simulink library "aerosimlib"  (Simulink 5.0)
values from neighbouring files (symbols this model uses):
  stdatm = [0 100 200 300 400 500 600 700 800 900 1000 1100 ... (4305 elements, 861x5)]    [stdatm.mat]
undefined symbols (not defined in the file or in its folder): AlphaBnd, b, BetaBnd, CDda, CDde, CDdf, CDdr, CDM, CDmin, CGempty, CGgross, CL0, CLa, CLalphadot, Clbeta, Clda, CLde, CLdf, Cldr, CLM, CLmind, Clp, CLq, Clr, Cm0, Cma, Cmalphadot, Cmde, Cmdf, CmM, Cmq, Cnbeta, Cnda, Cndr, Cnp, Cnr, CP, CT, CYbeta, CYda, CYdr, CYp, CYr, Displacement, dmy, Engine, EulerIni, FuelFlow, FuelIni, J, Jempty, Jeng, Jgross, Jprop, MAC, MAP, MAPLim, MassIni, MaxPower, mempty ... (+25)
libraries: aerosimlib x350, simulink3 x41
(part 9 of 10)

== system aerosimlib/FlightGear-Compatible/Complete Aircraft/CESSNA-182/Aerodynamics/Roll ==
  Control : Inport  PortDimensions=[4 1]
  WindAxesVel : Inport  Port=2  PortDimensions=[3 1]
  AngularRates : Inport  Port=3  PortDimensions=[3 1]
  2 : Gain  Gain=2  SaturateOnIntegerOverflow=on
  Cl aileron : Subsystem  BlockChoice=Value
      link override Value: Value=AC.Aerodynamics.Roll.ClDa
      settings: AttributesFormatString=%<BlockChoice>  TemplateBlock=aerosimlib/FlightGear-Compatible/Aerodynamics/Coefficient  MemberBlocks=Table,Value,Vector
  Cl beta : Subsystem  BlockChoice=Table
      link override Table: Table=AC.Aerodynamics.Roll.Clb
      link override Value: Value=AC.Aerodynamics.Lift.Basic.kCLge
      link override Vector: Vector=AC.Aerodynamics.Roll.Clb
      settings: AttributesFormatString=%<BlockChoice>  TemplateBlock=aerosimlib/FlightGear-Compatible/Aerodynamics/Coefficient  MemberBlocks=Table,Value,Vector
  Cl rudder : Subsystem  BlockChoice=Value
      link override Value: Value=AC.Aerodynamics.Roll.ClDr
      settings: AttributesFormatString=%<BlockChoice>  TemplateBlock=aerosimlib/FlightGear-Compatible/Aerodynamics/Coefficient  MemberBlocks=Table,Value,Vector
  Cl*b/(2V) : Product  Inputs=**/  SaturateOnIntegerOverflow=on  InputSameDT=on
  Clp : Subsystem  BlockChoice=Vector
      link override Value: Value=AC.Aerodynamics.Roll.Clp
      link override Vector: Vector=AC.Aerodynamics.Roll.Clp
      settings: AttributesFormatString=%<BlockChoice>  TemplateBlock=aerosimlib/FlightGear-Compatible/Aerodynamics/Coefficient  MemberBlocks=Table,Value,Vector
  Clp*p : Product  SaturateOnIntegerOverflow=on  InputSameDT=on
  Clr : Subsystem  BlockChoice=Vector
      link override Value: Value=AC.Aerodynamics.Side.CYdr
      link override Vector: Vector=AC.Aerodynamics.Roll.Clr
      settings: AttributesFormatString=%<BlockChoice>  TemplateBlock=aerosimlib/FlightGear-Compatible/Aerodynamics/Coefficient  MemberBlocks=Table,Value,Vector
  Clr*r : Product  SaturateOnIntegerOverflow=on  InputSameDT=on
  Demux : Demux
  Demux1 : Demux  Outputs=3
  Demux3 : Demux  Outputs=3
  Sum : Sum  SaturateOnIntegerOverflow=on  InputSameDT=on
  Sum1 : Sum  Inputs=++++  SaturateOnIntegerOverflow=on  InputSameDT=on
  Terminator2 : Terminator
  Terminator3 : Terminator
  Terminator4 : Terminator
  Wing span : Constant  Value=AC.Metrics.WingSpan
  Cl : Outport
  wires:
  Demux3/3 -> Clr*r/2
  Demux3/1 -> Clp*p/2
  Clp*p/1 -> Sum/1
  Clr*r/1 -> Sum/2
  Clr/1(Coeff) -> Clr*r/1
  Clp/1(Coeff) -> Clp*p/1
  Sum1/1 -> Cl/1
  AngularRates/1 -> Demux3/1
  Control/1 -> Demux/1
  WindAxesVel/1 -> Demux1/1
  Wing span/1 -> Cl*b/(2V)/2
  2/1 -> Cl*b/(2V)/3
  Sum/1 -> Cl*b/(2V)/1
  Demux1/1 -> 2/1
  Demux1/2 -> Cl beta/1(RowParam)
  Demux/3 -> Cl aileron/1(RowParam)
  Demux/4 -> Cl rudder/1(RowParam)
  Demux3/2 -> Terminator4/1
  Demux1/3 -> Clr/1(RowParam), Clp/1(RowParam), Cl beta/2(ColParam)
  Demux/1 -> Terminator2/1
  Demux/2 -> Terminator3/1
  Cl beta/1(Coeff) -> Sum1/1
  Cl aileron/1(Coeff) -> Sum1/2
  Cl rudder/1(Coeff) -> Sum1/3
  Cl*b/(2V)/1 -> Sum1/4

== system aerosimlib/FlightGear-Compatible/Complete Aircraft/CESSNA-182/Aerodynamics/Side ==
  Control : Inport  PortDimensions=[4 1]
  WindAxesVel : Inport  Port=2  PortDimensions=[3 1]
  AngularRates : Inport  Port=3  PortDimensions=[3 1]
  2 : Gain  Gain=2  SaturateOnIntegerOverflow=on
  CY aileron : Subsystem  BlockChoice=Value
      link override Value: Value=AC.Aerodynamics.Side.CYDa
      settings: AttributesFormatString=%<BlockChoice>  TemplateBlock=aerosimlib/FlightGear-Compatible/Aerodynamics/Coefficient  MemberBlocks=Table,Value,Vector
  CY beta : Subsystem  BlockChoice=Vector
      link override Value: Value=AC.Aerodynamics.Lift.Basic.kCLge
      link override Vector: Vector=AC.Aerodynamics.Side.CYb
      settings: AttributesFormatString=%<BlockChoice>  TemplateBlock=aerosimlib/FlightGear-Compatible/Aerodynamics/Coefficient  MemberBlocks=Table,Value,Vector
  CY rudder : Subsystem  BlockChoice=Value
      link override Value: Value=AC.Aerodynamics.Side.CYDr
      settings: AttributesFormatString=%<BlockChoice>  TemplateBlock=aerosimlib/FlightGear-Compatible/Aerodynamics/Coefficient  MemberBlocks=Table,Value,Vector
  CY*b/(2V) : Product  Inputs=**/  SaturateOnIntegerOverflow=on  InputSameDT=on
  CYb*b : Product  SaturateOnIntegerOverflow=on  InputSameDT=on
  CYp : Subsystem  BlockChoice=Vector
      link override Value: Value=AC.Aerodynamics.Side.CYp
      link override Vector: Vector=AC.Aerodynamics.Side.CYp
      settings: AttributesFormatString=%<BlockChoice>  TemplateBlock=aerosimlib/FlightGear-Compatible/Aerodynamics/Coefficient  MemberBlocks=Table,Value,Vector
  CYp*p : Product  SaturateOnIntegerOverflow=on  InputSameDT=on
  CYr : Subsystem  BlockChoice=Vector
      link override Value: Value=AC.Aerodynamics.Side.CYr
      link override Vector: Vector=AC.Aerodynamics.Side.CYr
      settings: AttributesFormatString=%<BlockChoice>  TemplateBlock=aerosimlib/FlightGear-Compatible/Aerodynamics/Coefficient  MemberBlocks=Table,Value,Vector
  CYr*r : Product  SaturateOnIntegerOverflow=on  InputSameDT=on
  Demux : Demux
  Demux1 : Demux  Outputs=3
  Demux3 : Demux  Outputs=3
  Sum : Sum  SaturateOnIntegerOverflow=on  InputSameDT=on
  Sum1 : Sum  Inputs=++++  SaturateOnIntegerOverflow=on  InputSameDT=on
  Terminator2 : Terminator
  Terminator3 : Terminator
  Terminator4 : Terminator
  Wing span : Constant  Value=AC.Metrics.WingSpan
  CY : Outport
  wires:
  Demux3/3 -> CYr*r/2
  Demux3/1 -> CYp*p/2
  CYr*r/1 -> Sum/2
  CYr/1(Coeff) -> CYr*r/1
  CYp*p/1 -> Sum/1
  CYp/1(Coeff) -> CYp*p/1
  Demux1/2 -> CYb*b/2
  CYb*b/1 -> Sum1/1
  CY beta/1(Coeff) -> CYb*b/1
  CY*b/(2V)/1 -> Sum1/4
  CY rudder/1(Coeff) -> Sum1/3
  CY aileron/1(Coeff) -> Sum1/2
  Demux/2 -> Terminator3/1
  Demux/1 -> Terminator2/1
  Demux1/3 -> CYr/1(RowParam), CYp/1(RowParam), CY beta/1(RowParam)
  Demux3/2 -> Terminator4/1
  Demux/4 -> CY rudder/1(RowParam)
  Demux/3 -> CY aileron/1(RowParam)
  Demux1/1 -> 2/1
  Sum/1 -> CY*b/(2V)/1
  2/1 -> CY*b/(2V)/3
  Wing span/1 -> CY*b/(2V)/2
  WindAxesVel/1 -> Demux1/1
  Control/1 -> Demux/1
  AngularRates/1 -> Demux3/1
  Sum1/1 -> CY/1

== system aerosimlib/FlightGear-Compatible/Complete Aircraft/CESSNA-182/Aerodynamics/Yaw ==
  Control : Inport  PortDimensions=[4 1]
  WindAxesVel : Inport  Port=2  PortDimensions=[3 1]
  AngularRates : Inport  Port=3  PortDimensions=[3 1]
  2 : Gain  Gain=2  SaturateOnIntegerOverflow=on
  Cn aileron : Subsystem  BlockChoice=Vector
      link override Value: Value=AC.Aerodynamics.Yaw.Cnda
      link override Vector: Vector=AC.Aerodynamics.Yaw.CnDa
      settings: AttributesFormatString=%<BlockChoice>  TemplateBlock=aerosimlib/FlightGear-Compatible/Aerodynamics/Coefficient  MemberBlocks=Table,Value,Vector
  Cn beta : Subsystem  BlockChoice=Vector
      link override Value: Value=AC.Aerodynamics.Lift.Basic.kCLge
      link override Vector: Vector=AC.Aerodynamics.Yaw.Cnb
      settings: AttributesFormatString=%<BlockChoice>  TemplateBlock=aerosimlib/FlightGear-Compatible/Aerodynamics/Coefficient  MemberBlocks=Table,Value,Vector
  Cn rudder : Subsystem  BlockChoice=Vector
      link override Value: Value=AC.Aerodynamics.Yaw.Cndr
      link override Vector: Vector=AC.Aerodynamics.Yaw.CnDr
      settings: AttributesFormatString=%<BlockChoice>  TemplateBlock=aerosimlib/FlightGear-Compatible/Aerodynamics/Coefficient  MemberBlocks=Table,Value,Vector
  Cn*b/(2V) : Product  Inputs=**/  SaturateOnIntegerOverflow=on  InputSameDT=on
  Cnb*b{,1..4} (5 alike) : Product  SaturateOnIntegerOverflow=on  InputSameDT=on
  Cnp : Subsystem  BlockChoice=Vector
      link override Value: Value=AC.Aerodynamics.Yaw.Cnp
      link override Vector: Vector=AC.Aerodynamics.Yaw.Cnp
      settings: AttributesFormatString=%<BlockChoice>  TemplateBlock=aerosimlib/FlightGear-Compatible/Aerodynamics/Coefficient  MemberBlocks=Table,Value,Vector
  Cnr : Subsystem  BlockChoice=Vector
      link override Value: Value=AC.Aerodynamics.Yaw.Cnr
      link override Vector: Vector=AC.Aerodynamics.Yaw.Cnr
      settings: AttributesFormatString=%<BlockChoice>  TemplateBlock=aerosimlib/FlightGear-Compatible/Aerodynamics/Coefficient  MemberBlocks=Table,Value,Vector
  Demux : Demux
  Demux1 : Demux  Outputs=3
  Demux3 : Demux  Outputs=3
  Sum : Sum  SaturateOnIntegerOverflow=on  InputSameDT=on
  Sum1 : Sum  Inputs=++++  SaturateOnIntegerOverflow=on  InputSameDT=on
  Terminator2 : Terminator
  Terminator3 : Terminator
  Terminator4 : Terminator
  Wing span : Constant  Value=AC.Metrics.WingSpan
  Cn : Outport
  wires:
  Demux3/3 -> Cnb*b4/2
  Demux3/1 -> Cnb*b3/2
  Demux/4 -> Cnb*b2/2
  Demux/3 -> Cnb*b1/2
  Cnb*b2/1 -> Sum1/3
  Cnb*b1/1 -> Sum1/2
  Cnb*b3/1 -> Sum/1
  Cnb*b4/1 -> Sum/2
  Cnr/1(Coeff) -> Cnb*b4/1
  Cnp/1(Coeff) -> Cnb*b3/1
  Cn rudder/1(Coeff) -> Cnb*b2/1
  Cn aileron/1(Coeff) -> Cnb*b1/1
  Demux1/2 -> Cnb*b/2
  Cn beta/1(Coeff) -> Cnb*b/1
  Cnb*b/1 -> Sum1/1
  Cn*b/(2V)/1 -> Sum1/4
  Demux/2 -> Terminator3/1
  Demux/1 -> Terminator2/1
  Demux1/3 -> Cnp/1(RowParam), Cnr/1(RowParam), Cn rudder/1(RowParam), Cn aileron/1(RowParam), Cn beta/1(RowParam)
  Demux3/2 -> Terminator4/1
  Demux1/1 -> 2/1
  Sum/1 -> Cn*b/(2V)/1
  2/1 -> Cn*b/(2V)/3
  Wing span/1 -> Cn*b/(2V)/2
  WindAxesVel/1 -> Demux1/1
  Control/1 -> Demux/1
  AngularRates/1 -> Demux3/1
  Sum1/1 -> Cn/1

== system aerosimlib/FlightGear-Compatible/Complete Aircraft/CESSNA-310/Aerodynamics/Drag ==
  Control : Inport  PortDimensions=[4 1]
  WindAxesVel : Inport  Port=2  PortDimensions=[3 1]
  Gear : Inport  Port=3  PortDimensions=1
  CD alpha : Subsystem  BlockChoice=Vector
      link override Table: Table=AC.Aerodynamics.Drag.Basic.CDwbh
      link override Value: Value=AC.Aerodynamics.Lift.Basic.kCLge
      link override Vector: Vector=AC.Aerodynamics.Drag.CDalpha
      settings: AttributesFormatString=%<BlockChoice>  TemplateBlock=aerosimlib/FlightGear-Compatible/Aerodynamics/Coefficient  MemberBlocks=Table,Value,Vector
  CD beta : Subsystem  BlockChoice=Value
      link override Value: Value=AC.Aerodynamics.Drag.CDbeta
      settings: AttributesFormatString=%<BlockChoice>  TemplateBlock=aerosimlib/FlightGear-Compatible/Aerodynamics/Coefficient  MemberBlocks=Table,Value,Vector
  CD elevator : Subsystem  BlockChoice=Value
      link override Value: Value=AC.Aerodynamics.Drag.CDDe
      settings: AttributesFormatString=%<BlockChoice>  TemplateBlock=aerosimlib/FlightGear-Compatible/Aerodynamics/Coefficient  MemberBlocks=Table,Value,Vector
  CD flap : Subsystem  BlockChoice=Vector
      link override Table: Table=AC.Aerodynamics.Drag.CDDf
      link override Value: Value=AC.Aerodynamics.Lift.Basic.kCLge
      link override Vector: Vector=AC.Aerodynamics.Drag.CDDf
      settings: AttributesFormatString=%<BlockChoice>  TemplateBlock=aerosimlib/FlightGear-Compatible/Aerodynamics/Coefficient  MemberBlocks=Table,Value,Vector
  CD gear : Subsystem  BlockChoice=Value
      link override Value: Value=AC.Aerodynamics.Drag.CDgear
      settings: AttributesFormatString=%<BlockChoice>  TemplateBlock=aerosimlib/FlightGear-Compatible/Aerodynamics/Coefficient  MemberBlocks=Table,Value,Vector
  CDo : Constant  Value=AC.Aerodynamics.Drag.CDo.Data
  Demux : Demux
  Demux1 : Demux  Outputs=3
  Sum : Sum  SaturateOnIntegerOverflow=on  InputSameDT=on
  Sum1 : Sum  Inputs=+++++  SaturateOnIntegerOverflow=on  InputSameDT=on
  Terminator : Terminator
  Terminator1 : Terminator
  Terminator5 : Terminator
  CD : Outport
  wires:
  Gear/1 -> CD gear/1(RowParam)
  CD gear/1(Coeff) -> Sum1/5
  Demux/2 -> CD elevator/1(RowParam)
  WindAxesVel/1 -> Demux1/1
  Control/1 -> Demux/1
  Demux/3 -> Terminator/1
  Demux/4 -> Terminator1/1
  Demux1/3 -> CD alpha/1(RowParam)
  CD alpha/1(Coeff) -> Sum/1
  CD flap/1(Coeff) -> Sum/2
  Sum/1 -> Sum1/1
  CDo/1 -> Sum1/2
  CD elevator/1(Coeff) -> Sum1/3
  Sum1/1 -> CD/1
  Demux1/1 -> Terminator5/1
  Demux1/2 -> CD beta/1(RowParam)
  Demux/1 -> CD flap/1(RowParam)
  CD beta/1(Coeff) -> Sum1/4

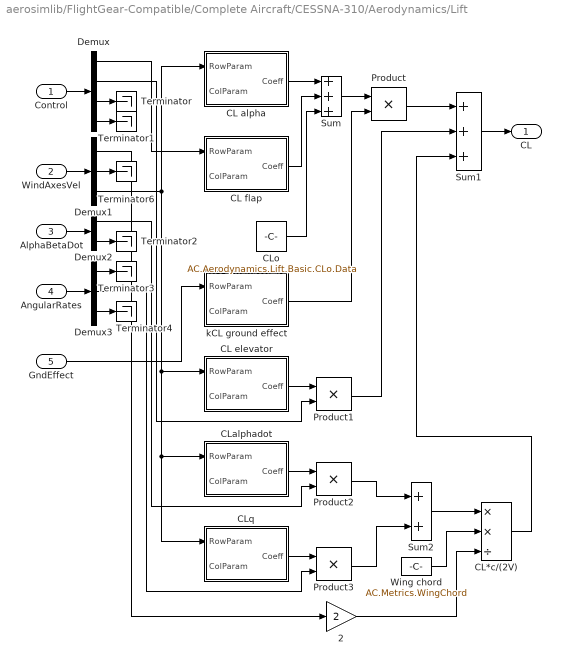
== system aerosimlib/FlightGear-Compatible/Complete Aircraft/CESSNA-310/Aerodynamics/Lift ==
  Control : Inport  PortDimensions=[4 1]
  WindAxesVel : Inport  Port=2  PortDimensions=[3 1]
  AlphaBetaDot : Inport  Port=3  PortDimensions=[2 1]
  AngularRates : Inport  Port=4  PortDimensions=[3 1]
  GndEffect : Inport  Port=5  PortDimensions=1
  2 : Gain  Gain=2  SaturateOnIntegerOverflow=on
  CL alpha : Subsystem  BlockChoice=Vector
      link override Table: Table=AC.Aerodynamics.Lift.Basic.CLalpha
      link override Value: Value=AC.Aerodynamics.Lift.Basic.kCLge
      link override Vector: Vector=AC.Aerodynamics.Lift.Basic.CLalpha
      settings: AttributesFormatString=%<BlockChoice>  TemplateBlock=aerosimlib/FlightGear-Compatible/Aerodynamics/Coefficient  MemberBlocks=Table,Value,Vector
  CL elevator : Subsystem  BlockChoice=Vector
      link override Value: Value=AC.Aerodynamics.Lift.CLDe
      link override Vector: Vector=AC.Aerodynamics.Lift.CLDe
      settings: AttributesFormatString=%<BlockChoice>  TemplateBlock=aerosimlib/FlightGear-Compatible/Aerodynamics/Coefficient  MemberBlocks=Table,Value,Vector
  CL flap : Subsystem  BlockChoice=Vector
      link override Value: Value=AC.Aerodynamics.Lift.Basic.kCLge
      link override Vector: Vector=AC.Aerodynamics.Lift.Basic.CLDf
      settings: AttributesFormatString=%<BlockChoice>  TemplateBlock=aerosimlib/FlightGear-Compatible/Aerodynamics/Coefficient  MemberBlocks=Table,Value,Vector
  CL*c/(2V) : Product  Inputs=**/  SaturateOnIntegerOverflow=on  InputSameDT=on
  CLalphadot : Subsystem  BlockChoice=Vector
      link override Value: Value=AC.Aerodynamics.Lift.CLadot
      link override Vector: Vector=AC.Aerodynamics.Lift.CLadot
      settings: AttributesFormatString=%<BlockChoice>  TemplateBlock=aerosimlib/FlightGear-Compatible/Aerodynamics/Coefficient  MemberBlocks=Table,Value,Vector
  CLo : Constant  Value=AC.Aerodynamics.Lift.Basic.CLo.Data
  CLq : Subsystem  BlockChoice=Vector
      link override Value: Value=AC.Aerodynamics.Lift.CLq
      link override Vector: Vector=AC.Aerodynamics.Lift.CLq
      settings: AttributesFormatString=%<BlockChoice>  TemplateBlock=aerosimlib/FlightGear-Compatible/Aerodynamics/Coefficient  MemberBlocks=Table,Value,Vector
  Demux : Demux
  Demux1 : Demux  Outputs=3
  Demux2 : Demux  Outputs=2
  Demux3 : Demux  Outputs=3
  Product{,1..3} (4 alike) : Product  SaturateOnIntegerOverflow=on  InputSameDT=on
  Sum : Sum  Inputs=+++  SaturateOnIntegerOverflow=on  InputSameDT=on
  Sum1 : Sum  Inputs=+++  SaturateOnIntegerOverflow=on  InputSameDT=on
  Sum2 : Sum  SaturateOnIntegerOverflow=on  InputSameDT=on
  Terminator{,1..4,6} (6 alike) : Terminator
  Wing chord : Constant  Value=AC.Metrics.WingChord
  kCL ground effect : Subsystem  BlockChoice=Vector
      link override Value: Value=AC.Aerodynamics.Lift.Basic.kCLge
      link override Vector: Vector=AC.Aerodynamics.Lift.Basic.kCLge
      settings: AttributesFormatString=%<BlockChoice>  TemplateBlock=aerosimlib/FlightGear-Compatible/Aerodynamics/Coefficient  MemberBlocks=Table,Value,Vector
  CL : Outport
  wires:
  Demux3/2 -> Product3/2
  Demux2/1 -> Product2/2
  Demux/2 -> Product1/2
  Product1/1 -> Sum1/2
  Product2/1 -> Sum2/1
  Product3/1 -> Sum2/2
  CLq/1(Coeff) -> Product3/1
  CLalphadot/1(Coeff) -> Product2/1
  CL elevator/1(Coeff) -> Product1/1
  CLo/1 -> Sum/3
  CL*c/(2V)/1 -> Sum1/3
  Sum2/1 -> CL*c/(2V)/1
  Wing chord/1 -> CL*c/(2V)/2
  2/1 -> CL*c/(2V)/3
  GndEffect/1 -> kCL ground effect/1(RowParam)
  Demux1/2 -> Terminator6/1
  Demux1/1 -> 2/1
  Sum1/1 -> CL/1
  Product/1 -> Sum1/1
  kCL ground effect/1(Coeff) -> Product/2
  Sum/1 -> Product/1
  CL flap/1(Coeff) -> Sum/2
  CL alpha/1(Coeff) -> Sum/1
  Demux3/3 -> Terminator4/1
  Demux3/1 -> Terminator3/1
  Demux2/2 -> Terminator2/1
  Demux1/3 -> CLq/1(RowParam), CLalphadot/1(RowParam), CL elevator/1(RowParam), CL alpha/1(RowParam)
  Demux/4 -> Terminator1/1
  Demux/3 -> Terminator/1
  Demux/1 -> CL flap/1(RowParam)
  AngularRates/1 -> Demux3/1
  AlphaBetaDot/1 -> Demux2/1
  Control/1 -> Demux/1
  WindAxesVel/1 -> Demux1/1

== system aerosimlib/FlightGear-Compatible/Complete Aircraft/CESSNA-310/Aerodynamics/Pitch ==
  Control : Inport  PortDimensions=[4 1]
  WindAxesVel : Inport  Port=2  PortDimensions=[3 1]
  AlphaBetaDot : Inport  Port=3  PortDimensions=[2 1]
  AngularRates : Inport  Port=4  PortDimensions=[3 1]
  2 : Gain  Gain=2  SaturateOnIntegerOverflow=on
  Cm alpha : Subsystem  BlockChoice=Value
      link override Table: Table=AC.Aerodynamics.Lift.Basic.CLwbh
      link override Value: Value=AC.Aerodynamics.Pitch.Cmalpha
      link override Vector: Vector=AC.Aerodynamics.Pitch.Cmalpha
      settings: AttributesFormatString=%<BlockChoice>  TemplateBlock=aerosimlib/FlightGear-Compatible/Aerodynamics/Coefficient  MemberBlocks=Table,Value,Vector
  Cm elevator : Subsystem  BlockChoice=Value
      link override Value: Value=AC.Aerodynamics.Pitch.CmDe
      link override Vector: Vector=AC.Aerodynamics.Pitch.CmDe
      settings: AttributesFormatString=%<BlockChoice>  TemplateBlock=aerosimlib/FlightGear-Compatible/Aerodynamics/Coefficient  MemberBlocks=Table,Value,Vector
  Cm flap : Subsystem  BlockChoice=Vector
      link override Value: Value=AC.Aerodynamics.Lift.Basic.kCLge
      link override Vector: Vector=AC.Aerodynamics.Pitch.CmDf
      settings: AttributesFormatString=%<BlockChoice>  TemplateBlock=aerosimlib/FlightGear-Compatible/Aerodynamics/Coefficient  MemberBlocks=Table,Value,Vector
  Cm*c/(2V) : Product  Inputs=**/  SaturateOnIntegerOverflow=on  InputSameDT=on
  Cmalphadot : Subsystem  BlockChoice=Value
      link override Value: Value=AC.Aerodynamics.Pitch.Cmadot
      link override Vector: Vector=AC.Aerodynamics.Pitch.Cmadot
      settings: AttributesFormatString=%<BlockChoice>  TemplateBlock=aerosimlib/FlightGear-Compatible/Aerodynamics/Coefficient  MemberBlocks=Table,Value,Vector
  Cmo : Constant  Value=AC.Aerodynamics.Pitch.Cmo.Data
  Cmq : Subsystem  BlockChoice=Value
      link override Value: Value=AC.Aerodynamics.Pitch.Cmq
      link override Vector: Vector=AC.Aerodynamics.Pitch.Cmq
      settings: AttributesFormatString=%<BlockChoice>  TemplateBlock=aerosimlib/FlightGear-Compatible/Aerodynamics/Coefficient  MemberBlocks=Table,Value,Vector
  Demux : Demux
  Demux1 : Demux  Outputs=3
  Demux2 : Demux  Outputs=2
  Demux3 : Demux  Outputs=3
  Sum1 : Sum  Inputs=+++++  SaturateOnIntegerOverflow=on  InputSameDT=on
  Sum2 : Sum  SaturateOnIntegerOverflow=on  InputSameDT=on
  Terminator{,1..4,6} (6 alike) : Terminator
  Wing chord : Constant  Value=AC.Metrics.WingChord
  Cm : Outport
  wires:
  Cm elevator/1(Coeff) -> Sum1/4
  Cm alpha/1(Coeff) -> Sum1/1
  Cm*c/(2V)/1 -> Sum1/5
  Cmo/1 -> Sum1/3
  Cm flap/1(Coeff) -> Sum1/2
  Demux1/3 -> Cm alpha/1(RowParam)
  Demux1/1 -> 2/1
  Demux/1 -> Cm flap/1(RowParam)
  WindAxesVel/1 -> Demux1/1
  Control/1 -> Demux/1
  AlphaBetaDot/1 -> Demux2/1
  AngularRates/1 -> Demux3/1
  Demux/3 -> Terminator/1
  Demux/4 -> Terminator1/1
  Demux2/2 -> Terminator2/1
  Demux3/1 -> Terminator3/1
  Demux3/3 -> Terminator4/1
  Sum1/1 -> Cm/1
  Demux1/2 -> Terminator6/1
  2/1 -> Cm*c/(2V)/3
  Wing chord/1 -> Cm*c/(2V)/2
  Sum2/1 -> Cm*c/(2V)/1
  Demux/2 -> Cm elevator/1(RowParam)
  Cmalphadot/1(Coeff) -> Sum2/1
  Cmq/1(Coeff) -> Sum2/2
  Demux2/1 -> Cmalphadot/1(RowParam)
  Demux3/2 -> Cmq/1(RowParam)

== system aerosimlib/FlightGear-Compatible/Complete Aircraft/CESSNA-310/Aerodynamics/Roll ==
  Control : Inport  PortDimensions=[4 1]
  WindAxesVel : Inport  Port=2  PortDimensions=[3 1]
  AngularRates : Inport  Port=3  PortDimensions=[3 1]
  2 : Gain  Gain=2  SaturateOnIntegerOverflow=on
  Cl aileron : Subsystem  BlockChoice=Value
      link override Value: Value=AC.Aerodynamics.Roll.ClDa
      settings: AttributesFormatString=%<BlockChoice>  TemplateBlock=aerosimlib/FlightGear-Compatible/Aerodynamics/Coefficient  MemberBlocks=Table,Value,Vector
  Cl beta : Subsystem  BlockChoice=Vector
      link override Table: Table=AC.Aerodynamics.Roll.Clbeta
      link override Value: Value=AC.Aerodynamics.Lift.Basic.kCLge
      link override Vector: Vector=AC.Aerodynamics.Roll.Clbeta
      settings: AttributesFormatString=%<BlockChoice>  TemplateBlock=aerosimlib/FlightGear-Compatible/Aerodynamics/Coefficient  MemberBlocks=Table,Value,Vector
  Cl rudder : Subsystem  BlockChoice=Value
      link override Value: Value=AC.Aerodynamics.Roll.Cldr
      settings: AttributesFormatString=%<BlockChoice>  TemplateBlock=aerosimlib/FlightGear-Compatible/Aerodynamics/Coefficient  MemberBlocks=Table,Value,Vector
  Cl*b/(2V) : Product  Inputs=**/  SaturateOnIntegerOverflow=on  InputSameDT=on
  Clp : Subsystem  BlockChoice=Value
      link override Value: Value=AC.Aerodynamics.Roll.Clp
      link override Vector: Vector=AC.Aerodynamics.Roll.Clp
      settings: AttributesFormatString=%<BlockChoice>  TemplateBlock=aerosimlib/FlightGear-Compatible/Aerodynamics/Coefficient  MemberBlocks=Table,Value,Vector
  Clr : Subsystem  BlockChoice=Value
      link override Value: Value=AC.Aerodynamics.Roll.Clr
      link override Vector: Vector=AC.Aerodynamics.Roll.Clr
      settings: AttributesFormatString=%<BlockChoice>  TemplateBlock=aerosimlib/FlightGear-Compatible/Aerodynamics/Coefficient  MemberBlocks=Table,Value,Vector
  Demux : Demux
  Demux1 : Demux  Outputs=3
  Demux3 : Demux  Outputs=3
  Sum : Sum  SaturateOnIntegerOverflow=on  InputSameDT=on
  Sum1 : Sum  Inputs=++++  SaturateOnIntegerOverflow=on  InputSameDT=on
  Terminator2 : Terminator
  Terminator3 : Terminator
  Terminator4 : Terminator
  Wing span : Constant  Value=AC.Metrics.WingSpan
  Cl : Outport
  wires:
  Clr/1(Coeff) -> Sum/2
  Clp/1(Coeff) -> Sum/1
  Sum1/1 -> Cl/1
  AngularRates/1 -> Demux3/1
  Control/1 -> Demux/1
  WindAxesVel/1 -> Demux1/1
  Wing span/1 -> Cl*b/(2V)/2
  2/1 -> Cl*b/(2V)/3
  Sum/1 -> Cl*b/(2V)/1
  Demux1/1 -> 2/1
  Demux1/2 -> Cl beta/1(RowParam)
  Demux/3 -> Cl aileron/1(RowParam)
  Demux/4 -> Cl rudder/1(RowParam)
  Demux3/2 -> Terminator4/1
  Demux/1 -> Terminator2/1
  Demux/2 -> Terminator3/1
  Cl beta/1(Coeff) -> Sum1/1
  Cl aileron/1(Coeff) -> Sum1/2
  Cl rudder/1(Coeff) -> Sum1/3
  Cl*b/(2V)/1 -> Sum1/4
  Demux3/1 -> Clp/1(RowParam)
  Demux3/3 -> Clr/1(RowParam)

== system aerosimlib/FlightGear-Compatible/Complete Aircraft/CESSNA-310/Aerodynamics/Side ==
  Control : Inport  PortDimensions=[4 1]
  WindAxesVel : Inport  Port=2  PortDimensions=[3 1]
  AngularRates : Inport  Port=3  PortDimensions=[3 1]
  2 : Gain  Gain=2  SaturateOnIntegerOverflow=on
  CY beta : Subsystem  BlockChoice=Vector
      link override Value: Value=AC.Aerodynamics.Lift.Basic.kCLge
      link override Vector: Vector=AC.Aerodynamics.Side.CYbeta
      settings: AttributesFormatString=%<BlockChoice>  TemplateBlock=aerosimlib/FlightGear-Compatible/Aerodynamics/Coefficient  MemberBlocks=Table,Value,Vector
  CY rudder : Subsystem  BlockChoice=Value
      link override Value: Value=AC.Aerodynamics.Side.CYDr
      settings: AttributesFormatString=%<BlockChoice>  TemplateBlock=aerosimlib/FlightGear-Compatible/Aerodynamics/Coefficient  MemberBlocks=Table,Value,Vector
  CY*b/(2V) : Product  Inputs=**/  SaturateOnIntegerOverflow=on  InputSameDT=on
  CYp : Subsystem  BlockChoice=Value
      link override Value: Value=AC.Aerodynamics.Side.CYp
      link override Vector: Vector=AC.Aerodynamics.Side.CYp
      settings: AttributesFormatString=%<BlockChoice>  TemplateBlock=aerosimlib/FlightGear-Compatible/Aerodynamics/Coefficient  MemberBlocks=Table,Value,Vector
  CYr : Subsystem  BlockChoice=Value
      link override Value: Value=AC.Aerodynamics.Side.CYr
      link override Vector: Vector=AC.Aerodynamics.Side.CYr
      settings: AttributesFormatString=%<BlockChoice>  TemplateBlock=aerosimlib/FlightGear-Compatible/Aerodynamics/Coefficient  MemberBlocks=Table,Value,Vector
  Demux : Demux
  Demux1 : Demux  Outputs=3
  Demux3 : Demux  Outputs=3
  Sum : Sum  SaturateOnIntegerOverflow=on  InputSameDT=on
  Sum1 : Sum  Inputs=++++  SaturateOnIntegerOverflow=on  InputSameDT=on
  Terminator2 : Terminator
  Terminator3 : Terminator
  Terminator4 : Terminator
  Wing span : Constant  Value=AC.Metrics.WingSpan
  CY : Outport
  wires:
  Demux3/3 -> CYr/1(RowParam)
  CYr/1(Coeff) -> Sum/2
  CYp/1(Coeff) -> Sum/1
  CY*b/(2V)/1 -> Sum1/4
  CY rudder/1(Coeff) -> Sum1/3
  Demux/2 -> Terminator3/1
  Demux/1 -> Terminator2/1
  Demux3/2 -> Terminator4/1
  Demux/4 -> CY rudder/1(RowParam)
  Demux1/1 -> 2/1
  Sum/1 -> CY*b/(2V)/1
  2/1 -> CY*b/(2V)/3
  Wing span/1 -> CY*b/(2V)/2
  WindAxesVel/1 -> Demux1/1
  Control/1 -> Demux/1
  AngularRates/1 -> Demux3/1
  Sum1/1 -> CY/1
  CY beta/1(Coeff) -> Sum1/1
  Demux1/2 -> CY beta/1(RowParam)
  Demux3/1 -> CYp/1(RowParam)

== system aerosimlib/FlightGear-Compatible/Complete Aircraft/CESSNA-310/Aerodynamics/Yaw ==
  Control : Inport  PortDimensions=[4 1]
  WindAxesVel : Inport  Port=2  PortDimensions=[3 1]
  AngularRates : Inport  Port=3  PortDimensions=[3 1]
  2 : Gain  Gain=2  SaturateOnIntegerOverflow=on
  Cn aileron : Subsystem  BlockChoice=Value
      link override Value: Value=AC.Aerodynamics.Yaw.CnDa
      link override Vector: Vector=AC.Aerodynamics.Yaw.CnDa
      settings: AttributesFormatString=%<BlockChoice>  TemplateBlock=aerosimlib/FlightGear-Compatible/Aerodynamics/Coefficient  MemberBlocks=Table,Value,Vector
  Cn beta : Subsystem  BlockChoice=Value
      link override Value: Value=AC.Aerodynamics.Yaw.Cnbeta
      link override Vector: Vector=AC.Aerodynamics.Yaw.Cnb
      settings: AttributesFormatString=%<BlockChoice>  TemplateBlock=aerosimlib/FlightGear-Compatible/Aerodynamics/Coefficient  MemberBlocks=Table,Value,Vector
  Cn rudder : Subsystem  BlockChoice=Value
      link override Value: Value=AC.Aerodynamics.Yaw.CnDr
      link override Vector: Vector=AC.Aerodynamics.Yaw.CnDr
      settings: AttributesFormatString=%<BlockChoice>  TemplateBlock=aerosimlib/FlightGear-Compatible/Aerodynamics/Coefficient  MemberBlocks=Table,Value,Vector
  Cn*b/(2V) : Product  Inputs=**/  SaturateOnIntegerOverflow=on  InputSameDT=on
  Cnp : Subsystem  BlockChoice=Value
      link override Value: Value=AC.Aerodynamics.Yaw.Cnp
      link override Vector: Vector=AC.Aerodynamics.Yaw.Cnp
      settings: AttributesFormatString=%<BlockChoice>  TemplateBlock=aerosimlib/FlightGear-Compatible/Aerodynamics/Coefficient  MemberBlocks=Table,Value,Vector
  Cnr : Subsystem  BlockChoice=Value
      link override Value: Value=AC.Aerodynamics.Yaw.Cnr
      link override Vector: Vector=AC.Aerodynamics.Yaw.Cnr
      settings: AttributesFormatString=%<BlockChoice>  TemplateBlock=aerosimlib/FlightGear-Compatible/Aerodynamics/Coefficient  MemberBlocks=Table,Value,Vector
  Demux : Demux
  Demux1 : Demux  Outputs=3
  Demux3 : Demux  Outputs=3
  Sum : Sum  SaturateOnIntegerOverflow=on  InputSameDT=on
  Sum1 : Sum  Inputs=++++  SaturateOnIntegerOverflow=on  InputSameDT=on
  Terminator2 : Terminator
  Terminator3 : Terminator
  Terminator4 : Terminator
  Wing span : Constant  Value=AC.Metrics.WingSpan
  Cn : Outport
  wires:
  Demux/4 -> Cn rudder/1(RowParam)
  Cn aileron/1(Coeff) -> Sum1/2
  Cnr/1(Coeff) -> Sum/2
  Cnp/1(Coeff) -> Sum/1
  Cn rudder/1(Coeff) -> Sum1/3
  Cn*b/(2V)/1 -> Sum1/4
  Demux/2 -> Terminator3/1
  Demux/1 -> Terminator2/1
  Demux3/2 -> Terminator4/1
  Demux1/1 -> 2/1
  Sum/1 -> Cn*b/(2V)/1
  2/1 -> Cn*b/(2V)/3
  Wing span/1 -> Cn*b/(2V)/2
  WindAxesVel/1 -> Demux1/1
  Control/1 -> Demux/1
  AngularRates/1 -> Demux3/1
  Sum1/1 -> Cn/1
  Demux/3 -> Cn aileron/1(RowParam)
  Cn beta/1(Coeff) -> Sum1/1
  Demux1/2 -> Cn beta/1(RowParam)
  Demux3/1 -> Cnp/1(RowParam)
  Demux3/3 -> Cnr/1(RowParam)

== system aerosimlib/FlightGear-Compatible/Propulsion/Engine/Piston/AirFlow Model ==
  MAP : Inport
  RPM : Inport  Port=2
  rho : Inport  Port=3
  p : Inport  Port=4
  1/2 : Gain  Gain=1/2  SaturateOnIntegerOverflow=on
  Displacement : Constant  Value=Disp/(100)^3
  Product : Product  SaturateOnIntegerOverflow=on  InputSameDT=on
  Product1 : Product  Inputs=3  SaturateOnIntegerOverflow=on  InputSameDT=on
  Product2 : Product  Inputs=**/  SaturateOnIntegerOverflow=on  InputSameDT=on
  Volumetric eff : Constant  Value=VolEff
  rot/sec : Gain  Gain=1/60  SaturateOnIntegerOverflow=on
  AirFlow : Outport
  wires:
  Product1/1 -> AirFlow/1
  Product2/1 -> Product1/3
  p/1 -> Product2/3
  MAP/1 -> Product2/2
  rho/1 -> Product2/1
  Volumetric eff/1 -> Product1/2
  1/2/1 -> Product1/1
  Product/1 -> 1/2/1
  Displacement/1 -> Product/2
  rot/sec/1 -> Product/1
  RPM/1 -> rot/sec/1

== system aerosimlib/FlightGear-Compatible/Propulsion/Engine/Piston/FG Piston Engine ==
  Thr : Inport  PortDimensions=1  DataType=double
  Mix : Inport  Port=2  PortDimensions=1  DataType=double
  Omega : Inport  Port=3  PortDimensions=1  DataType=double
  p : Inport  Port=4  PortDimensions=1  DataType=double
  T : Inport  Port=5  PortDimensions=1  DataType=double
  rho : Inport  Port=6  PortDimensions=1  DataType=double
  AirFlow Model : aerosimlib/FlightGear-Compatible/Propulsion/Engine/Piston/AirFlow Model  VolEff=0.8  Disp=Eng.Param.Displacement
  Engine torque : Product  Inputs=*/  SaturateOnIntegerOverflow=on  InputSameDT=on
  Engine  BSFC : Product  Inputs=*/  SaturateOnIntegerOverflow=on  InputSameDT=on
  FuelFlow Model : aerosimlib/FlightGear-Compatible/Propulsion/Engine/Piston/FuelFlow Model  pSL=pSL
  Intake Model : aerosimlib/FlightGear-Compatible/Propulsion/Engine/Piston/Intake Model  MAPLim=Eng.Param.MAPLim  pSL=pSL
  Power Model : aerosimlib/FlightGear-Compatible/Propulsion/Engine/Piston/Power Model  TSL=TSL  MaxPower=Eng.Param.MaxPower  Mixture=[14.7/1.6 10 11 12 13 14 15 16 17 18 19 20 14.7/0.6]  PowerMixCor=[78 86 93 98 100 99 96.4 92.5 88 83 78.5 74 58]
  rad/s 2 RPM : aerosimlib/Unit Conversion/Angular velocity/rad//s 2 RPM
  MAP : Outport
  AirFlow : Outport  Port=2
  FuelFlow : Outport  Port=3
  BSFC : Outport  Port=4
  Power : Outport  Port=5
  Torque : Outport  Port=6
  wires:
  Power Model/1 -> Engine torque/1, Engine  BSFC/2, Power/1
  FuelFlow Model/2 -> FuelFlow/1, Engine  BSFC/1
  Mix/1 -> FuelFlow Model/1
  rho/1 -> AirFlow Model/3
  T/1 -> Power Model/3
  FuelFlow Model/1 -> Power Model/4
  AirFlow Model/1 -> AirFlow/1, FuelFlow Model/3
  rad/s 2 RPM/1 -> Power Model/2, AirFlow Model/2
  Intake Model/1 -> MAP/1, Power Model/1, AirFlow Model/1
  Omega/1 -> Engine torque/2, rad/s 2 RPM/1
  Engine  BSFC/1 -> BSFC/1
  Engine torque/1 -> Torque/1
  Thr/1 -> Intake Model/1
  p/1 -> AirFlow Model/4, FuelFlow Model/2, Intake Model/2

== system aerosimlib/FlightGear-Compatible/Propulsion/Engine/Piston/FuelFlow Model ==
  Mix : Inport
  p : Inport  Port=2
  AirFlow : Inport  Port=3
  Gain : Gain  Gain=1.3  SaturateOnIntegerOverflow=on
  Product : Product  Inputs=**/  SaturateOnIntegerOverflow=on  InputSameDT=on
  Product1 : Product  Inputs=**/  SaturateOnIntegerOverflow=on  InputSameDT=on
  Sea-level pressure : Constant  Value=pSL
  coef : Constant  Value=14.7
  EquivRatio : Outport
  FuelFlow : Outport  Port=2
  wires:
  Product1/1 -> FuelFlow/1
  coef/1 -> Product1/3
  AirFlow/1 -> Product1/2
  Product/1 -> Product1/1, EquivRatio/1
  p/1 -> Product/3
  Sea-level pressure/1 -> Product/2
  Gain/1 -> Product/1
  Mix/1 -> Gain/1

== system aerosimlib/FlightGear-Compatible/Propulsion/Engine/Piston/Intake Model ==
  Thr : Inport  PortDimensions=1  DataType=double
  p : Inport  Port=2  PortDimensions=1  DataType=double
  Get MAP Altitude : Product  Inputs=**/  SaturateOnIntegerOverflow=on  InputSameDT=on
  Get MAP Sea-level : Product  SaturateOnIntegerOverflow=on  InputSameDT=on
  MAP max : Constant  Value=MAPLim(2)
  MAP min : Constant  Value=MAPLim(1)
  Saturation : Saturate  UpperLimit=MAPLim(2)  LowerLimit=MAPLim(1)
  Sum : Sum  Inputs=|+-  SaturateOnIntegerOverflow=on  InputSameDT=on
  Sum1 : Sum  Inputs=|++  SaturateOnIntegerOverflow=on  InputSameDT=on
  p ambient : Constant  Value=pSL
  MAP : Outport
  wires:
  Get MAP Altitude/1 -> MAP/1
  p ambient/1 -> Get MAP Altitude/3
  p/1 -> Get MAP Altitude/2
  Saturation/1 -> Get MAP Altitude/1
  MAP max/1 -> Sum/1
  Thr/1 -> Get MAP Sea-level/1
  MAP min/1 -> Sum/2, Sum1/2
  Sum/1 -> Get MAP Sea-level/2
  Get MAP Sea-level/1 -> Sum1/1
  Sum1/1 -> Saturation/1

== system aerosimlib/FlightGear-Compatible/Propulsion/Engine/Piston/Power Model ==
  MAP : Inport
  RPM : Inport  Port=2
  T : Inport  Port=3
  EquivRatio : Inport  Port=4
  Gain : Gain  Gain=1/100  SaturateOnIntegerOverflow=on
  Gain1 : Gain  Gain=1/100  SaturateOnIntegerOverflow=on
  K2F : aerosimlib/Unit Conversion/Temperature/K2F
  K2F1 : aerosimlib/Unit Conversion/Temperature/K2F
  Look-Up Table : Lookup  InputValues=Mixture  OutputValues=PowerMixCor  SaturateOnIntegerOverflow=on
  Math Function : Math  Operator=square
  MaxPower : Constant  Value=MaxPower
  Pa2inHg : aerosimlib/Unit Conversion/Pressure/Pa2inHg
  Product{,1..3} (4 alike) : Product  SaturateOnIntegerOverflow=on  InputSameDT=on
  Product4 : Product  Inputs=3  SaturateOnIntegerOverflow=on  InputSameDT=on
  Product5 : Product  Inputs=*/  SaturateOnIntegerOverflow=on  InputSameDT=on
  Sum : Sum  Inputs=++-+  SaturateOnIntegerOverflow=on  InputSameDT=on
  Sum1 : Sum  Inputs=|+-  SaturateOnIntegerOverflow=on  InputSameDT=on
  T ambient : Constant  Value=TSL
  coef1 : Constant  Value=6e-9
  coef2 : Constant  Value=8e-4
  coef3 : Constant
  coef4 : Constant  Value=7/120
  coef5 : Constant  Value=14.7
  Power : Outport
  wires:
  coef5/1 -> Product5/1
  EquivRatio/1 -> Product5/2
  Product5/1 -> Look-Up Table/1
  Product4/1 -> Power/1
  MaxPower/1 -> Product4/3
  Gain/1 -> Product4/2
  Gain1/1 -> Product4/1
  Sum/1 -> Gain1/1
  Look-Up Table/1 -> Gain/1
  Product3/1 -> Sum/4
  coef4/1 -> Product3/2
  Sum1/1 -> Product3/1
  RPM/1 -> Product/2
  Pa2inHg/1 -> Product/1
  K2F/1 -> Sum1/2
  K2F1/1 -> Sum1/1
  T ambient/1 -> K2F1/1
  T/1 -> K2F/1
  coef3/1 -> Sum/3
  Product2/1 -> Sum/2
  Product1/1 -> Sum/1
  coef2/1 -> Product2/2
  coef1/1 -> Product1/2
  Math Function/1 -> Product1/1
  Product/1 -> Product2/1, Math Function/1
  MAP/1 -> Pa2inHg/1

== system aerosimlib/FlightGear-Compatible/Propulsion/Thruster/Propeller/FG Fixed-Pitch Propeller ==
  note: Sources
  note: Compute advance ratio
  note: Compute thrust force
  note: Interpolate propeller coefficients
  note: Compute torque
  Airspeed : Inport  PortDimensions=1  DataType=double
  rho : Inport  Port=2  PortDimensions=1  DataType=double
  Omega : Inport  Port=3  PortDimensions=1  DataType=double
  1/pi^2 : Math  Operator=pow
  1/pi^3 : Math  Operator=pow
  Advance Ratio : Product  Inputs=**//  SaturateOnIntegerOverflow=on  InputSameDT=on
  Coeff of Power : Lookup  InputValues=Thr.Param.CoefPower(:,1)  OutputValues=Thr.Param.CoefPower(:,2)  SaturateOnIntegerOverflow=on
  Coeff of Thrust : Lookup  InputValues=Thr.Param.CoefThrust(:,1)  OutputValues=Thr.Param.CoefThrust(:,2)  SaturateOnIntegerOverflow=on
  Gain : Gain  Gain=4  SaturateOnIntegerOverflow=on
  Gain1 : Gain  Gain=-4  SaturateOnIntegerOverflow=on
  Mux : Mux  Inputs=3
  Omega^2 : Math  Operator=square
  Pi : Constant  Value=pi
  Prop Radius : Constant  Value=Thr.Param.Diameter/2
  R^4 : Math  Operator=pow
  R^5 : Math  Operator=pow
  Thrust : Product  Inputs=5  SaturateOnIntegerOverflow=on  InputSameDT=on
  Torque : Product  Inputs=5  SaturateOnIntegerOverflow=on  InputSameDT=on
  exp : Constant  Value=-3
  exp1 : Constant  Value=4
  exp2 : Constant  Value=5
  exp3 : Constant  Value=-2
  Fprop : Outport
  Mprop : Outport  Port=2
  PropCoeff : Outport  Port=3
  wires:
  exp3/1 -> 1/pi^2/2
  Coeff of Power/1 -> Mux/3, Torque/5
  Airspeed/1 -> Advance Ratio/2
  rho/1 -> Torque/2, Thrust/2
  Omega/1 -> Advance Ratio/3, Omega^2/1
  Pi/1 -> Advance Ratio/1, 1/pi^2/1, 1/pi^3/1
  Prop Radius/1 -> Advance Ratio/4, R^4/1, R^5/1
  Advance Ratio/1 -> Mux/1, Coeff of Power/1, Coeff of Thrust/1
  Omega^2/1 -> Torque/4, Thrust/4
  exp/1 -> 1/pi^3/2
  1/pi^2/1 -> Gain/1
  1/pi^3/1 -> Gain1/1
  exp1/1 -> R^4/2
  R^4/1 -> Thrust/3
  exp2/1 -> R^5/2
  R^5/1 -> Torque/3
  Gain/1 -> Thrust/1
  Gain1/1 -> Torque/1
  Coeff of Thrust/1 -> Mux/2, Thrust/5
  Thrust/1 -> Fprop/1
  Torque/1 -> Mprop/1
  Mux/1 -> PropCoeff/1

== system aerosimlib/FlightGear-Compatible/Propulsion/Thruster/Propeller/FG Variable-Pitch Propeller ==
  note: Sources
  note: Compute advance ratio
  note: Compute thrust force
  note: Interpolate propeller coefficients
  note: Compute torque
  Airspeed : Inport  PortDimensions=1  DataType=double
  rho : Inport  Port=2  PortDimensions=1  DataType=double
  Omega : Inport  Port=3  PortDimensions=1  DataType=double
  Pitch : Inport  Port=4  PortDimensions=1  DataType=double
  1/pi^2 : Math  Operator=pow
  1/pi^3 : Math  Operator=pow
  Advance Ratio : Product  Inputs=**//  SaturateOnIntegerOverflow=on  InputSameDT=on
  Coeff of Power : Lookup2D  RowIndex=Thr.Param.CoefPower(2:end,1)  ColumnIndex=Thr.Param.CoefPower(1,2:end)  OutputValues=Thr.Param.CoefPower(2:end,2:end)  SaturateOnIntegerOverflow=on  InputSameDT=on
  Coeff of Thrust : Lookup2D  RowIndex=Thr.Param.CoefThrust(2:end,1)  ColumnIndex=Thr.Param.CoefThrust(1,2:end)  OutputValues=Thr.Param.CoefThrust(2:end,2:end)  SaturateOnIntegerOverflow=on  InputSameDT=on
  Gain : Gain  Gain=4  SaturateOnIntegerOverflow=on
  Gain1 : Gain  Gain=-4  SaturateOnIntegerOverflow=on
  Mux : Mux  Inputs=3
  Omega^2 : Math  Operator=square
  Pi : Constant  Value=pi
  Prop Radius : Constant  Value=Thr.Param.Diameter/2
  R^4 : Math  Operator=pow
  R^5 : Math  Operator=pow
  Thrust : Product  Inputs=5  SaturateOnIntegerOverflow=on  InputSameDT=on
  Torque : Product  Inputs=5  SaturateOnIntegerOverflow=on  InputSameDT=on
  exp : Constant  Value=-3
  exp1 : Constant  Value=4
  exp2 : Constant  Value=5
  exp3 : Constant  Value=-2
  Fprop : Outport
  Mprop : Outport  Port=2
  PropCoeff : Outport  Port=3
  wires:
  Pitch/1 -> Coeff of Power/2, Coeff of Thrust/2
  exp3/1 -> 1/pi^2/2
  Coeff of Power/1 -> Mux/3, Torque/5
  Airspeed/1 -> Advance Ratio/2
  rho/1 -> Torque/2, Thrust/2
  Omega/1 -> Advance Ratio/3, Omega^2/1
  Pi/1 -> Advance Ratio/1, 1/pi^2/1, 1/pi^3/1
  Prop Radius/1 -> Advance Ratio/4, R^4/1, R^5/1
  Advance Ratio/1 -> Coeff of Power/1, Mux/1, Coeff of Thrust/1
  Omega^2/1 -> Torque/4, Thrust/4
  exp/1 -> 1/pi^3/2
  1/pi^2/1 -> Gain/1
  1/pi^3/1 -> Gain1/1
  exp1/1 -> R^4/2
  R^4/1 -> Thrust/3
  exp2/1 -> R^5/2
  R^5/1 -> Torque/3
  Gain/1 -> Thrust/1
  Gain1/1 -> Torque/1
  Coeff of Thrust/1 -> Mux/2, Thrust/5
  Thrust/1 -> Fprop/1
  Torque/1 -> Mprop/1
  Mux/1 -> PropCoeff/1

== system aerosimlib/FlightGear-Compatible/Complete Aircraft/CESSNA-172/Aerodynamics/Drag/CD alpha ==
  RowParam : Inport
  ColParam : Inport  Port=2
  Table : aerosimlib/FlightGear-Compatible/Aerodynamics/Table  Table=AC.Aerodynamics.Drag.Basic.CDwbh
  Coeff : Outport
  wires:
  Table/1 -> Coeff/1
  ColParam/1 -> Table/2
  RowParam/1 -> Table/1

== system aerosimlib/FlightGear-Compatible/Complete Aircraft/CESSNA-172/Aerodynamics/Drag/CD beta ==
  RowParam : Inport
  ColParam : Inport  Port=2
  Value : aerosimlib/FlightGear-Compatible/Aerodynamics/Value  Value=AC.Aerodynamics.Drag.CDbeta
  term2 : Terminator
  Coeff : Outport
  wires:
  ColParam/1 -> term2/1
  Value/1 -> Coeff/1
  RowParam/1 -> Value/1

== system aerosimlib/FlightGear-Compatible/Complete Aircraft/CESSNA-172/Aerodynamics/Drag/CD elevator ==
  RowParam : Inport
  ColParam : Inport  Port=2
  Value : aerosimlib/FlightGear-Compatible/Aerodynamics/Value  Value=AC.Aerodynamics.Drag.CDDe
  term2 : Terminator
  Coeff : Outport
  wires:
  ColParam/1 -> term2/1
  Value/1 -> Coeff/1
  RowParam/1 -> Value/1

== system aerosimlib/FlightGear-Compatible/Complete Aircraft/CESSNA-172/Aerodynamics/Drag/CD flap ==
  RowParam : Inport
  ColParam : Inport  Port=2
  Vector : aerosimlib/FlightGear-Compatible/Aerodynamics/Vector  Vector=AC.Aerodynamics.Drag.Basic.CDDf
  term2 : Terminator
  Coeff : Outport
  wires:
  ColParam/1 -> term2/1
  Vector/1 -> Coeff/1
  RowParam/1 -> Vector/1

== system aerosimlib/FlightGear-Compatible/Complete Aircraft/CESSNA-172/Aerodynamics/Drag/kCD ground effect ==
  RowParam : Inport
  ColParam : Inport  Port=2
  Vector : aerosimlib/FlightGear-Compatible/Aerodynamics/Vector  Vector=AC.Aerodynamics.Drag.Basic.kCDge
  term2 : Terminator
  Coeff : Outport
  wires:
  ColParam/1 -> term2/1
  Vector/1 -> Coeff/1
  RowParam/1 -> Vector/1

== system aerosimlib/FlightGear-Compatible/Complete Aircraft/CESSNA-172/Aerodynamics/Lift/CL alpha ==
  RowParam : Inport
  ColParam : Inport  Port=2
  Table : aerosimlib/FlightGear-Compatible/Aerodynamics/Table  Table=AC.Aerodynamics.Lift.Basic.CLwbh
  Coeff : Outport
  wires:
  RowParam/1 -> Table/1
  ColParam/1 -> Table/2
  Table/1 -> Coeff/1

== system aerosimlib/FlightGear-Compatible/Complete Aircraft/CESSNA-172/Aerodynamics/Lift/CL elevator ==
  RowParam : Inport
  ColParam : Inport  Port=2
  Value : aerosimlib/FlightGear-Compatible/Aerodynamics/Value  Value=AC.Aerodynamics.Lift.CLDe
  term2 : Terminator
  Coeff : Outport
  wires:
  RowParam/1 -> Value/1
  Value/1 -> Coeff/1
  ColParam/1 -> term2/1

== system aerosimlib/FlightGear-Compatible/Complete Aircraft/CESSNA-172/Aerodynamics/Lift/CL flap ==
  RowParam : Inport
  ColParam : Inport  Port=2
  Vector : aerosimlib/FlightGear-Compatible/Aerodynamics/Vector  Vector=AC.Aerodynamics.Lift.Basic.CLDf
  term2 : Terminator
  Coeff : Outport
  wires:
  RowParam/1 -> Vector/1
  Vector/1 -> Coeff/1
  ColParam/1 -> term2/1

== system aerosimlib/FlightGear-Compatible/Complete Aircraft/CESSNA-172/Aerodynamics/Lift/CLalphadot ==
  RowParam : Inport
  ColParam : Inport  Port=2
  Value : aerosimlib/FlightGear-Compatible/Aerodynamics/Value  Value=AC.Aerodynamics.Lift.CLadot
  term2 : Terminator
  Coeff : Outport
  wires:
  RowParam/1 -> Value/1
  Value/1 -> Coeff/1
  ColParam/1 -> term2/1

== system aerosimlib/FlightGear-Compatible/Complete Aircraft/CESSNA-172/Aerodynamics/Lift/CLq ==
  RowParam : Inport
  ColParam : Inport  Port=2
  Value : aerosimlib/FlightGear-Compatible/Aerodynamics/Value  Value=AC.Aerodynamics.Lift.CLq
  term2 : Terminator
  Coeff : Outport
  wires:
  RowParam/1 -> Value/1
  Value/1 -> Coeff/1
  ColParam/1 -> term2/1

== system aerosimlib/FlightGear-Compatible/Complete Aircraft/CESSNA-172/Aerodynamics/Lift/kCL ground effect ==
  RowParam : Inport
  ColParam : Inport  Port=2
  Vector : aerosimlib/FlightGear-Compatible/Aerodynamics/Vector  Vector=AC.Aerodynamics.Lift.Basic.kCLge
  term2 : Terminator
  Coeff : Outport
  wires:
  RowParam/1 -> Vector/1
  Vector/1 -> Coeff/1
  ColParam/1 -> term2/1

== system aerosimlib/FlightGear-Compatible/Complete Aircraft/CESSNA-172/Aerodynamics/Pitch/Cm alpha ==
  RowParam : Inport
  ColParam : Inport  Port=2
  Value : aerosimlib/FlightGear-Compatible/Aerodynamics/Value  Value=AC.Aerodynamics.Pitch.Cmalpha
  term2 : Terminator
  Coeff : Outport
  wires:
  RowParam/1 -> Value/1
  Value/1 -> Coeff/1
  ColParam/1 -> term2/1

== system aerosimlib/FlightGear-Compatible/Complete Aircraft/CESSNA-172/Aerodynamics/Pitch/Cm elevator ==
  RowParam : Inport
  ColParam : Inport  Port=2
  Value : aerosimlib/FlightGear-Compatible/Aerodynamics/Value  Value=AC.Aerodynamics.Pitch.Cmde
  term2 : Terminator
  Coeff : Outport
  wires:
  RowParam/1 -> Value/1
  Value/1 -> Coeff/1
  ColParam/1 -> term2/1

== system aerosimlib/FlightGear-Compatible/Complete Aircraft/CESSNA-172/Aerodynamics/Pitch/Cm flap ==
  RowParam : Inport
  ColParam : Inport  Port=2
  Vector : aerosimlib/FlightGear-Compatible/Aerodynamics/Vector  Vector=AC.Aerodynamics.Pitch.Cmdf
  term2 : Terminator
  Coeff : Outport
  wires:
  RowParam/1 -> Vector/1
  Vector/1 -> Coeff/1
  ColParam/1 -> term2/1

== system aerosimlib/FlightGear-Compatible/Complete Aircraft/CESSNA-172/Aerodynamics/Pitch/Cmalphadot ==
  RowParam : Inport
  ColParam : Inport  Port=2
  Value : aerosimlib/FlightGear-Compatible/Aerodynamics/Value  Value=AC.Aerodynamics.Pitch.Cmadot
  term2 : Terminator
  Coeff : Outport
  wires:
  RowParam/1 -> Value/1
  Value/1 -> Coeff/1
  ColParam/1 -> term2/1

== system aerosimlib/FlightGear-Compatible/Complete Aircraft/CESSNA-172/Aerodynamics/Pitch/Cmq ==
  RowParam : Inport
  ColParam : Inport  Port=2
  Value : aerosimlib/FlightGear-Compatible/Aerodynamics/Value  Value=AC.Aerodynamics.Pitch.Cmq
  term2 : Terminator
  Coeff : Outport
  wires:
  RowParam/1 -> Value/1
  Value/1 -> Coeff/1
  ColParam/1 -> term2/1

== system aerosimlib/FlightGear-Compatible/Complete Aircraft/CESSNA-172/Aerodynamics/Roll/Cl aileron ==
  RowParam : Inport
  ColParam : Inport  Port=2
  Value : aerosimlib/FlightGear-Compatible/Aerodynamics/Value  Value=AC.Aerodynamics.Roll.ClDa
  term2 : Terminator
  Coeff : Outport
  wires:
  RowParam/1 -> Value/1
  Value/1 -> Coeff/1
  ColParam/1 -> term2/1

== system aerosimlib/FlightGear-Compatible/Complete Aircraft/CESSNA-172/Aerodynamics/Roll/Cl beta ==
  RowParam : Inport
  ColParam : Inport  Port=2
  Vector : aerosimlib/FlightGear-Compatible/Aerodynamics/Vector  Vector=AC.Aerodynamics.Roll.Clb
  term2 : Terminator
  Coeff : Outport
  wires:
  RowParam/1 -> Vector/1
  Vector/1 -> Coeff/1
  ColParam/1 -> term2/1

== system aerosimlib/FlightGear-Compatible/Complete Aircraft/CESSNA-172/Aerodynamics/Roll/Cl rudder ==
  RowParam : Inport
  ColParam : Inport  Port=2
  Value : aerosimlib/FlightGear-Compatible/Aerodynamics/Value  Value=AC.Aerodynamics.Roll.Cldr
  term2 : Terminator
  Coeff : Outport
  wires:
  RowParam/1 -> Value/1
  Value/1 -> Coeff/1
  ColParam/1 -> term2/1

== system aerosimlib/FlightGear-Compatible/Complete Aircraft/CESSNA-172/Aerodynamics/Roll/Clp ==
  RowParam : Inport
  ColParam : Inport  Port=2
  Value : aerosimlib/FlightGear-Compatible/Aerodynamics/Value  Value=AC.Aerodynamics.Roll.Clp
  term2 : Terminator
  Coeff : Outport
  wires:
  RowParam/1 -> Value/1
  Value/1 -> Coeff/1
  ColParam/1 -> term2/1

== system aerosimlib/FlightGear-Compatible/Complete Aircraft/CESSNA-172/Aerodynamics/Roll/Clr ==
  RowParam : Inport
  ColParam : Inport  Port=2
  Table : aerosimlib/FlightGear-Compatible/Aerodynamics/Table  Table=AC.Aerodynamics.Roll.Clr
  Coeff : Outport
  wires:
  RowParam/1 -> Table/1
  ColParam/1 -> Table/2
  Table/1 -> Coeff/1

== system aerosimlib/FlightGear-Compatible/Complete Aircraft/CESSNA-172/Aerodynamics/Side/CY aileron ==
  RowParam : Inport
  ColParam : Inport  Port=2
  Value : aerosimlib/FlightGear-Compatible/Aerodynamics/Value  Value=AC.Aerodynamics.Side.CYda
  term2 : Terminator
  Coeff : Outport
  wires:
  RowParam/1 -> Value/1
  Value/1 -> Coeff/1
  ColParam/1 -> term2/1

== system aerosimlib/FlightGear-Compatible/Complete Aircraft/CESSNA-172/Aerodynamics/Side/CY beta ==
  RowParam : Inport
  ColParam : Inport  Port=2
  Table : aerosimlib/FlightGear-Compatible/Aerodynamics/Table  Table=AC.Aerodynamics.Side.CYb
  Coeff : Outport
  wires:
  RowParam/1 -> Table/1
  ColParam/1 -> Table/2
  Table/1 -> Coeff/1

== system aerosimlib/FlightGear-Compatible/Complete Aircraft/CESSNA-172/Aerodynamics/Side/CY rudder ==
  RowParam : Inport
  ColParam : Inport  Port=2
  Value : aerosimlib/FlightGear-Compatible/Aerodynamics/Value  Value=AC.Aerodynamics.Side.CYdr
  term2 : Terminator
  Coeff : Outport
  wires:
  RowParam/1 -> Value/1
  Value/1 -> Coeff/1
  ColParam/1 -> term2/1

== system aerosimlib/FlightGear-Compatible/Complete Aircraft/CESSNA-172/Aerodynamics/Side/CYp ==
  RowParam : Inport
  ColParam : Inport  Port=2
  Table : aerosimlib/FlightGear-Compatible/Aerodynamics/Table  Table=AC.Aerodynamics.Side.CYp
  Coeff : Outport
  wires:
  RowParam/1 -> Table/1
  ColParam/1 -> Table/2
  Table/1 -> Coeff/1

== system aerosimlib/FlightGear-Compatible/Complete Aircraft/CESSNA-172/Aerodynamics/Side/CYr ==
  RowParam : Inport
  ColParam : Inport  Port=2
  Table : aerosimlib/FlightGear-Compatible/Aerodynamics/Table  Table=AC.Aerodynamics.Side.CYr
  Coeff : Outport
  wires:
  RowParam/1 -> Table/1
  ColParam/1 -> Table/2
  Table/1 -> Coeff/1

== system aerosimlib/FlightGear-Compatible/Complete Aircraft/CESSNA-172/Aerodynamics/Yaw/Cn aileron ==
  RowParam : Inport
  ColParam : Inport  Port=2
  Value : aerosimlib/FlightGear-Compatible/Aerodynamics/Value  Value=AC.Aerodynamics.Yaw.Cnda
  term2 : Terminator
  Coeff : Outport
  wires:
  ColParam/1 -> term2/1
  Value/1 -> Coeff/1
  RowParam/1 -> Value/1

== system aerosimlib/FlightGear-Compatible/Complete Aircraft/CESSNA-172/Aerodynamics/Yaw/Cn beta ==
  RowParam : Inport
  ColParam : Inport  Port=2
  Vector : aerosimlib/FlightGear-Compatible/Aerodynamics/Vector  Vector=AC.Aerodynamics.Yaw.Cnb
  term2 : Terminator
  Coeff : Outport
  wires:
  ColParam/1 -> term2/1
  Vector/1 -> Coeff/1
  RowParam/1 -> Vector/1

== system aerosimlib/FlightGear-Compatible/Complete Aircraft/CESSNA-172/Aerodynamics/Yaw/Cn rudder ==
  RowParam : Inport
  ColParam : Inport  Port=2
  Value : aerosimlib/FlightGear-Compatible/Aerodynamics/Value  Value=AC.Aerodynamics.Yaw.Cndr
  term2 : Terminator
  Coeff : Outport
  wires:
  ColParam/1 -> term2/1
  Value/1 -> Coeff/1
  RowParam/1 -> Value/1
